simulink model "half_shaft"  (R2024a)
settings: Solver=VariableStepAuto  StartTime=0.0  StopTime=10.0  RelTol=1e-3
values from neighbouring files (symbols this model uses):
  drivetrain_gain = 10.5    [assignment_2.m]
  tors_stiff = 9000    [assignment_2.m]
settings Model: Creator=fjmo  LastModifiedBy=fjmo

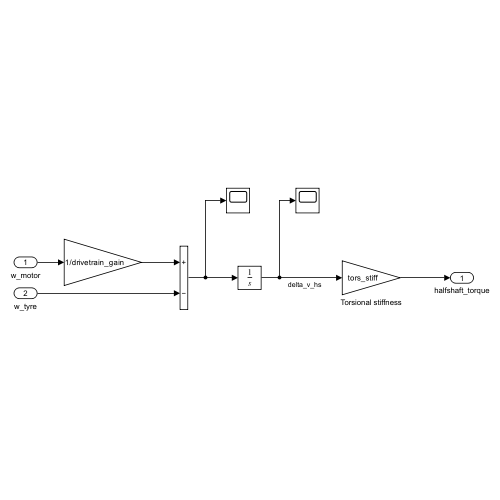
[thumbnail: Simulink's stored preview of the top-level diagram]
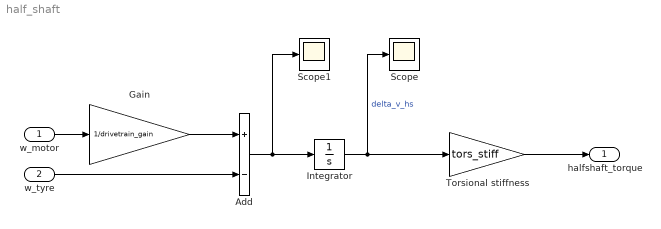
== system half_shaft ==
  w_motor : Inport
  w_tyre : Inport  Port=2
  Add : Sum  Inputs=+-
  Gain : Gain  Gain=1/drivetrain_gain
  Integrator : Integrator
  Scope : Scope
  Scope1 : Scope
  Torsional stiffness : Gain  Gain=tors_stiff
  halfshaft_torque : Outport
  wires:
  w_tyre/1 -> Add/2
  Integrator/1 -> Torsional stiffness/1, Scope/1  "delta_v_hs"
  Torsional stiffness/1 -> halfshaft_torque/1
  Add/1 -> Scope1/1, Integrator/1
  w_motor/1 -> Gain/1
  Gain/1 -> Add/1
